simulink model "EEE463_HardwareProject_final_design"  (R2024b)
settings: Solver=VariableStepAuto  StartTime=0.0  StopTime=10  RelTol=1e-3
libraries: spsDiodeLib x7, spsCurrentMeasurementLib x4, spsVoltageMeasurementLib x4, spsDCMachineLib x1, spsDCVoltageSourceLib x1, spsGroundLib x1, spsMosfetLib x1, slpidlib x1, simulink x1, spsSeriesRLCBranchLib x1, spsThreePhaseProgrammableVoltageSourceLib x1, spsThreePhaseVIMeasurementLib x1
settings Model: Creator=Asus  LastModifiedBy=pipil

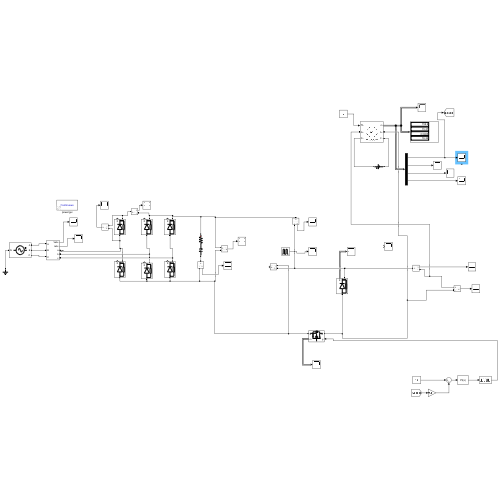
[thumbnail: Simulink's stored preview of the top-level diagram]
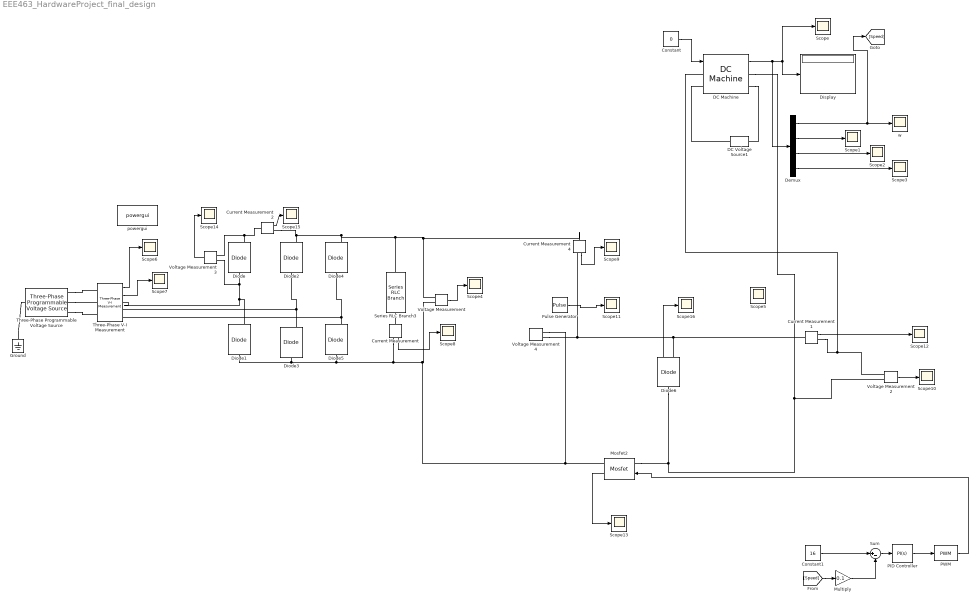
== system EEE463_HardwareProject_final_design ==
  Constant : Constant  Value=0
  Constant1 : Constant  Value=16
  Current Measurement{,1..2,4} (4 alike) : spsCurrentMeasurementLib/Current Measurement  PhasorSimulation=off  OutputType=Complex  PSBequivalent=0
  DC Machine : spsDCMachineLib/DC Machine  PresetModel=No  MechanicalLoad=Torque TL  FieldType=Wound  ShowDetailedParameters=on  MeasurementBus=off  RLa="[ 0.8  12.5e-3]"  RLf="[ 210  23]"  Laf=1.8  MachineConstant=Torque constant (N.m/A)  Ke=1.8  Kt=1.8  J=1  Bm=0.1  Tf=0.1  w0=1  Ifinit=0.590476190448228  TsPowergui=0  TsBlock=-1
  DC Voltage Source1 : spsDCVoltageSourceLib/DC Voltage Source  Amplitude=124  Measurements=None
  Demux : Demux
  Diode{,1..5} (6 alike) : spsDiodeLib/Diode  Ron=0.0325  Lon=0  Vf=0.98  IC=0  UseSnubber=0  Rs=500  Cs=250e-9  Measurements=on
  Diode6 : spsDiodeLib/Diode  Ron=0.217  Lon=0  Vf=1.3  IC=0  UseSnubber=0  Rs=500  Cs=250e-9  Measurements=on
  Display : Display
  Ground : spsGroundLib/Ground  LConnTagsString=a
  Mosfet2 : spsMosfetLib/Mosfet  Ron=0.15  Lon=0  Rd=0.01  Vfd=0  IC=0  Rs=1e5  Cs=inf  Measurements=on
  Multiply : Gain  Gain=0.1
  PID Controller : slpidlib/PID Controller  Controller=PI  Form=Parallel  TimeDomain=Continuous-time  UseExternalTs=off  SampleTime=-1  IntegratorMethod=Forward Euler  FilterMethod=Forward Euler  ControllerParametersSource=internal  P=0.01  I=0.02  UseKiTs=off  D=0  UseExternalDerivativeSource=off  N=100  UseFilter=on  TunerSelectOption=Transfer Function Based (PID Tuner App)  InitialConditionSource=internal  InitialConditionForIntegrator=0  InitialConditionForFilter=0  DifferentiatorICPrevScaledInput=0  ExternalReset=none  TrackingMode=off  Kt=1  LimitOutput=off  SatLimitsSource=internal  UpperSaturationLimit=inf  LowerSaturationLimit=-inf  LinearizeAsGain=on  AntiWindupMode=none  Kb=1  LimitIntegrator=off  UpperIntegratorSaturationLimit=inf  LowerIntegratorSaturationLimit=-inf  POutMin=[]  POutMax=[]  IOutMin=[]  IOutMax=[]  DOutMin=[]  DOutMax=[]  NOutMin=[]  NOutMax=[]  SumOutMin=[]  SumOutMax=[]  SaturationOutMin=[]  SaturationOutMax=[]  PParamMin=[]  PParamMax=[]  IParamMin=[]  IParamMax=[]  DParamMin=[]  DParamMax=[]  NParamMin=[]  NParamMax=[]  KbParamMin=[]  KbParamMax=[]  KtParamMin=[]  KtParamMax=[]  KbOutMin=[]  KbOutMax=[]  KtOutMin=[]  KtOutMax=[]  IntegratorOutMin=[]  IntegratorOutMax=[]  FilterOutMin=[]  FilterOutMax=[]  SumI1OutMin=[]  SumI1OutMax=[]  SumI2OutMin=[]  SumI2OutMax=[]  SumI3OutMin=[]  SumI3OutMax=[]  SumI4OutMin=[]  SumI4OutMax=[]  SumDOutMin=[]  SumDOutMax=[]  DifferentiatorOutMin=[]  DifferentiatorOutMax=[]  FilterDiffOutCoefMin=[]  FilterDiffOutCoefMax=[]  ReciprocalOutMin=[]  ReciprocalOutMax=[]  SumDenOutMin=[]  SumDenOutMax=[]  SumNumOutMin=[]  SumNumOutMax=[]  DivideOutMin=[]  DivideOutMax=[]  UdiffTsProdOutMin=[]  UdiffTsProdOutMax=[]  NTsProdOutMin=[]  NTsProdOutMax=[]  UintegralTsProdOutMin=[]  UintegralTsProdOutMax=[]  UngainTsProdOutMin=[]  UngainTsProdOutMax=[]  ClampingZeroOutDataTypeStr=Inherit: Inherit via back propagation  ClampingZeroOutMin=[]  ClampingZeroOutMax=[]  FilterDenConstantOutDataTypeStr=Inherit: Inherit via back propagation  FilterDenConstantOutMin=[]  FilterDenConstantOutMax=[]  PCopyOutDataTypeStr=Inherit: Inherit via back propagation  PCopyOutMin=[]  PCopyOutMax=[]  NCopyOutDataTypeStr=Inherit: Inherit via back propagation  NCopyOutMin=[]  NCopyOutMax=[]  IntegratorContinuousStateAttributes=''  IntegratorStateMustResolveToSignalObject=off  IntegratorRTWStateStorageClass=Auto  FilterContinuousStateAttributes=''  FilterStateMustResolveToSignalObject=off  FilterRTWStateStorageClass=Auto  ParallelPVariant=InternalParameters  IdealPVariant=Disabled  IVariant=InternalParameters  DVariant=Disabled  IntegratorVariant=Continuous  SatVariant=Disabled  AWVariant=Passthrough  PCopyVariant=Disabled  TRVariant=Disabled  FdbkBlocksVariant=Forward  IdealPFdbkVariant=Disabled  SatFdbkVariant=Disabled  DerivativeFilterVariant=Disabled  NVariant=Disabled  NCopyVariant=Disabled_SignalSpec  FilterICVariant=Disabled  IntegratorICVariant=InternalICs  ExternalResetVariant=Disabled  TRSumVariant=Passthrough  SumFdbkVariant=Disabled  SumVariant=Sum_PI  TsampFilterVariant=InternalTs  TsampNgainVariant=Passthrough  TsampIntegralVariant=Disabled_SignalSpec  ExternalSaturationOutDataTypeStr=Inherit: Same as second input  DerivativeSourceVariant=Disabled  PreIntVariant=InternalPreInt
  PWM : simulink/Discontinuities/PWM  DisableCoverage=on  Period=10e-4  InitialDelay=0  DisallowZeroDutyCycle=off  RunAtFixedTimeIntervals=off  SampleTime=0.1
  Pulse Generator : DiscretePulseGenerator  PulseType=Time based  Amplitude=5  Period=1/10000  PulseWidth=85
  Scope{,1..16} (17 alike) : Scope
  Series RLC Branch3 : spsSeriesRLCBranchLib/Series RLC Branch  LConnTagsString=__new0  RConnTagsString=__new0  BranchType=RC  Resistance=0.04  Inductance=1e-3  SetiL0=off  InitialCurrent=0  Capacitance=1000e-6  Setx0=off  InitialVoltage=0  Measurements=None
  Sum : Sum  Inputs=|+-
  Three-Phase Programmable Voltage Source : spsThreePhaseProgrammableVoltageSourceLib/Three-Phase Programmable Voltage Source  PositiveSequence="[150  0 50]"  VariationEntity=None  VariationType=Table of time-amplitude pairs  VariationTypeAlt=Step  VariationStep=0.5  VariationRate=10  VariationMagnitude=0.3  VariationFrequency=2  VariationTiming=[1 2]  VariationPhaseA=off  Amplitudes="[0.1  0.3  0.5  0.7  0.9 1]"  TimeValues="[0  0.2  0.4  0.6  0.8 0.9]"  HarmonicGeneration=off  HarmonicA=[3 0.2 -25 0]  HarmonicB=[2 0.15 35 2]  Timing="[0.05  3]"  BusType=swing  Pref=0  Qref=0  Qmin=-inf  Qmax=inf
  Three-Phase V-I Measurement : spsThreePhaseVIMeasurementLib/Three-Phase V-I Measurement  VoltageMeasurement=phase-to-phase  SetLabelV=off  LabelV=Vabc  Vpu=off  VpuLL=off  CurrentMeasurement=yes  SetLabelI=off  LabelI=Iabc  Ipu=off  Pbase=100e6  Vbase=500e3  OutputType=Complex  PhasorSimulation=off  PSBequivalent=0
  Voltage Measurement{,2..4} (4 alike) : spsVoltageMeasurementLib/Voltage Measurement  PhasorSimulation=off  OutputType=Complex  PSBequivalent=0
  powergui : sps_lib/powergui  Priority=1  SimulationMode=Continuous  SampleTime=50e-6  frequency=60  Iterations=50  frequencyindice=0  Pbase=100e6  ErrMax=1e-4  UnitsV=kV  UnitsW=MW  buscounter=0  FunctionMessages=off  echomessages=off  EnableUseOfTLC=off  CurrentSourceSwitches=off  DisableSnubberDevices=off  DisableRonSwitches=off  DisableVfSwitches=off  DisplayEquations=off  AutomaticDiscreteSolvers=off  SolverType=Tustin/Backward Euler (TBE)  Interpol=off  ExternalGateDelay=off  methode=off  Ts=100  x0status=blocks  SPID=on  SwTol=0  HookPort=off  NonlinearTolerance=1e-4  nMaxIteration=100  ContinueOnMaxIteration=off  RestoreLinks=warning  ResistiveCurrentMeasurement=off  Frange=[0:2:500]  Ylog=off  Xlog=on  ShowGrid=off  save=off  variable=ZData  structure=0  ZoomFFT=off  StartTime=0.0  cycles=1  DisplayStyle=1  fundamental=60  FreqAxis=off  MaxFrequency=1000  frequencyindicesteady=1  RmsSteady=1  display=off
  w : Scope
  wires:
  Three-Phase V-I Measurement/1 -> Scope6/1
  Voltage Measurement/1 -> Scope4/1
  Current Measurement/1 -> Scope8/1
  Three-Phase V-I Measurement/2 -> Scope7/1
  Current Measurement2/1 -> Scope15/1
  DC Machine/1 -> Demux/1, Scope/1, Display/1
  Voltage Measurement2/1 -> Scope10/1
  Demux/2 -> Scope1/1
  Demux/4 -> Scope3/1
  Current Measurement1/1 -> Scope12/1
  Constant/1 -> DC Machine/1
  Pulse Generator/1 -> Scope11/1
  Demux/3 -> Scope2/1
  Current Measurement4/1 -> Scope9/1
  Voltage Measurement3/1 -> Scope14/1
  Diode6/1 -> Scope16/1
  [Speed] -> Multiply/1
  Constant1/1 -> Sum/1
  Multiply/1 -> Sum/2
  Sum/1 -> PID Controller/1
  PID Controller/1 -> PWM/1
  PWM/1 -> Mosfet2/1
  Mosfet2/1 -> Scope13/1
  Demux/1 -> w/1, [Speed]
  connections:
  Diode4/RConn1 -- Current Measurement4/LConn1 -- Voltage Measurement/LConn1 -- Series RLC Branch3/LConn1 -- Current Measurement2/RConn1 -- Diode2/RConn1
  Voltage Measurement2/LConn2 -- DC Machine/RConn1 -- Mosfet2/LConn1 -- Diode6/LConn1
  Diode1/RConn1 -- Three-Phase V-I Measurement/RConn1 -- Voltage Measurement3/LConn1 -- Diode/LConn1
  Diode2/LConn1 -- Diode3/RConn1 -- Three-Phase V-I Measurement/RConn2
  Diode4/LConn1 -- Diode5/RConn1 -- Three-Phase V-I Measurement/RConn3
  Diode/RConn1 -- Voltage Measurement3/LConn2 -- Current Measurement2/LConn1
  Three-Phase Programmable Voltage Source/RConn2 -- Three-Phase V-I Measurement/LConn2
  Ground/LConn1 -- Three-Phase Programmable Voltage Source/LConn1
  Three-Phase Programmable Voltage Source/RConn1 -- Three-Phase V-I Measurement/LConn1
  Current Measurement/LConn1 -- Series RLC Branch3/RConn1
  Three-Phase Programmable Voltage Source/RConn3 -- Three-Phase V-I Measurement/LConn3
  Voltage Measurement2/LConn1 -- Current Measurement1/RConn1 -- DC Machine/LConn1
  DC Voltage Source1/RConn1 -- DC Machine/LConn2
  DC Machine/RConn2 -- DC Voltage Source1/LConn1
  Current Measurement1/LConn1 -- Voltage Measurement4/LConn1 -- Current Measurement4/RConn1 -- Diode6/RConn1
  Voltage Measurement4/LConn2 -- Mosfet2/RConn1 -- Current Measurement/RConn1 -- Diode5/LConn1 -- Diode1/LConn1 -- Diode3/LConn1 -- Voltage Measurement/LConn2
